simulink model "SUbsystem"  (R2025a)
settings: Solver=VariableStepAuto  StartTime=0.0  StopTime=30.0  RelTol=1e-3
InitFcn:
  | m = 0.111;
  | R = 0.015;
  | d = 0.03;
  | g = -9.8;
  | L = 1.0;
  | J = 9.99e-6;
settings Model: Creator=cruisemac  LastModifiedBy=cruisemac

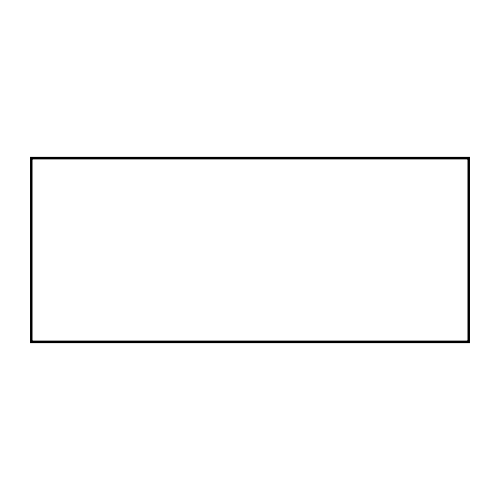
[thumbnail: Simulink's stored preview of the top-level diagram]
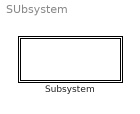
== system SUbsystem ==
  Subsystem : Subsystem

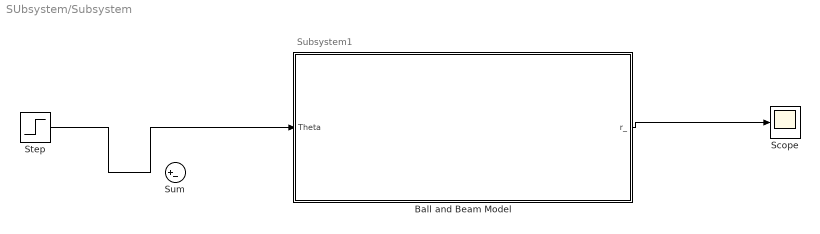
== system SUbsystem/Subsystem ==
  note: Subsystem1
  "Ball and Beam Model " : Subsystem
  Scope : Scope
      settings: ActiveDisplayYMinimum=-0.25011493002065088  ActiveDisplayYMaximum=2.2510343701858586
  Step : Step  Time=0  SampleTime=0
  Sum : Sum  Inputs=|+-
  wires:
  "Ball and Beam Model "/1(r_) -> Scope/1
  Step/1 -> "Ball and Beam Model "/1(Theta)

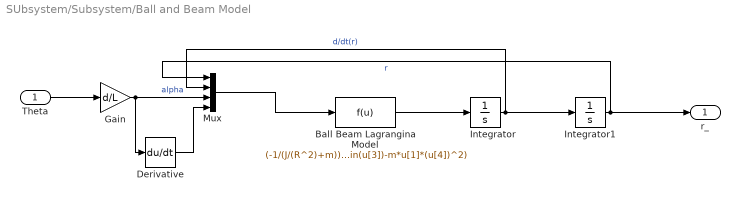
== system SUbsystem/Subsystem/Ball and Beam Model  ==
  Theta : Inport
  Ball Beam Lagrangina Model : Fcn  Expr=(-1/(J/(R^2)+m))*(m*g*sin(u[3])-m*u[1]*(u[4])^2)
  Derivative : Derivative
  Gain : Gain  Gain=d/L
  Integrator : Integrator
  Integrator1 : Integrator
  Mux : Mux
  r_ : Outport
  wires:
  Ball Beam Lagrangina Model/1 -> Integrator/1
  Gain/1 -> Derivative/1, Mux/3  "alpha"
  Integrator1/1 -> r_/1, Mux/1  "r"
  Integrator/1 -> Mux/2, Integrator1/1  "d/dt(r)"
  Mux/1 -> Ball Beam Lagrangina Model/1
  Derivative/1 -> Mux/4
  Theta/1 -> Gain/1
